simulink model "cordeuse"  (R2016b)
settings: Solver=VariableStepAuto  StartTime=0.0  StopTime=10.0  RelTol=1e-3
undefined symbols (not defined in the file): J, Ka, Kc, Kcorde, Ke, Kh, Km, Kr, R, r, Rp
libraries: simulink x1
settings Model: Creator=emiliendurif  LastModifiedBy=emiliendurif

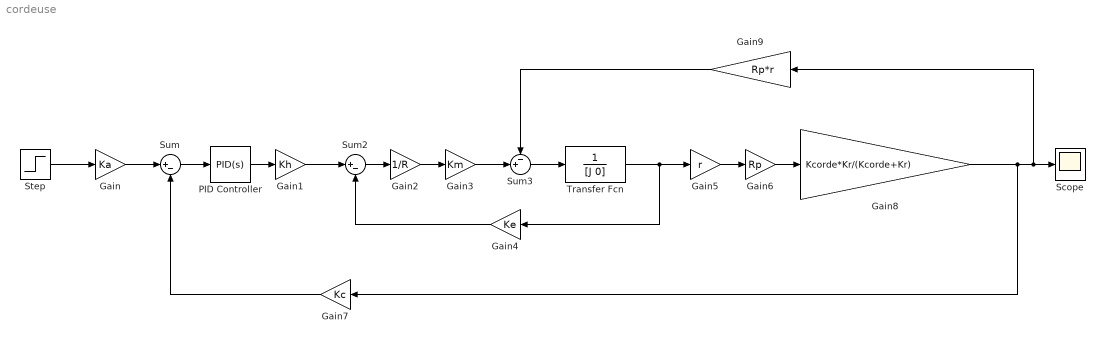
== system cordeuse ==
  Gain : Gain  Gain=Ka
  Gain1 : Gain  Gain=Kh
  Gain2 : Gain  Gain=1/R
  Gain3 : Gain  Gain=Km
  Gain4 : Gain  Gain=Ke
  Gain5 : Gain  Gain=r
  Gain6 : Gain  Gain=Rp
  Gain7 : Gain  Gain=Kc
  Gain8 : Gain  Gain=Kcorde*Kr/(Kcorde+Kr)
  Gain9 : Gain  Gain=Rp*r
  PID Controller : simulink/Continuous/PID Controller  Controller=PID  TimeDomain=Continuous-time  SampleTime=-1  IntegratorMethod=Forward Euler  FilterMethod=Forward Euler  Form=Parallel  UseFilter=on  ControllerParametersSource=internal  P=20  I=0  D=0  N=100  InitialConditionSource=internal  InitialConditionForIntegrator=0  InitialConditionForFilter=0  ExternalReset=none  LimitOutput=off  UpperSaturationLimit=inf  LowerSaturationLimit=-inf  LinearizeAsGain=on  AntiWindupMode=none  Kb=1  TrackingMode=off  Kt=1  PParamMin=[]  PParamMax=[]  IParamMin=[]  IParamMax=[]  DParamMin=[]  DParamMax=[]  NParamMin=[]  NParamMax=[]  KbParamMin=[]  KbParamMax=[]  KtParamMin=[]  KtParamMax=[]  POutMin=[]  POutMax=[]  IOutMin=[]  IOutMax=[]  DOutMin=[]  DOutMax=[]  NOutMin=[]  NOutMax=[]  KbOutMin=[]  KbOutMax=[]  KtOutMin=[]  KtOutMax=[]  IntegratorOutMin=[]  IntegratorOutMax=[]  FilterOutMin=[]  FilterOutMax=[]  SumOutMin=[]  SumOutMax=[]  SumI1OutMin=[]  SumI1OutMax=[]  SumI2OutMin=[]  SumI2OutMax=[]  SumI3OutMin=[]  SumI3OutMax=[]  SumDOutMin=[]  SumDOutMax=[]  SaturationOutMin=[]  SaturationOutMax=[]  IntegratorContinuousStateAttributes=''  IntegratorStateMustResolveToSignalObject=off  IntegratorRTWStateStorageClass=Auto  FilterContinuousStateAttributes=''  FilterStateMustResolveToSignalObject=off  FilterRTWStateStorageClass=Auto  DifferentiatorICPrevScaledInput=0  DifferentiatorOutMin=[]  DifferentiatorOutMax=[]
  Scope : Scope
  Step : Step  Time=0  After=200  SampleTime=0
  Sum : Sum  Inputs=|+-
  Sum2 : Sum  Inputs=|+-
  Sum3 : Sum  Inputs=-+|
  Transfer Fcn : TransferFcn  Denominator=[J 0]
  wires:
  PID Controller/1 -> Gain1/1
  Sum/1 -> PID Controller/1
  Gain/1 -> Sum/1
  Step/1 -> Gain/1
  Gain1/1 -> Sum2/1
  Sum2/1 -> Gain2/1
  Gain2/1 -> Gain3/1
  Gain4/1 -> Sum2/2
  Transfer Fcn/1 -> Gain4/1, Gain5/1
  Gain5/1 -> Gain6/1
  Gain7/1 -> Sum/2
  Gain3/1 -> Sum3/2
  Sum3/1 -> Transfer Fcn/1
  Gain6/1 -> Gain8/1
  Gain8/1 -> Gain7/1, Gain9/1, Scope/1
  Gain9/1 -> Sum3/1
